simulink model "PSK"  (R2020b)
settings: Solver=VariableStepAuto  StartTime=0.0  StopTime=10.0  RelTol=1e-3
settings Model: Creator=LENOVO  LastModifiedBy=LENOVO

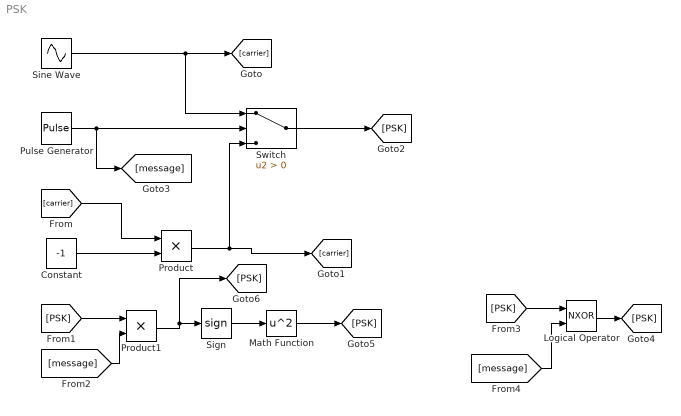
== system PSK ==
  Constant : Constant  Value=-1
  Logical Operator : Logic  Operator=NXOR  AllPortsSameDT=off  OutDataTypeStr=boolean
  Math Function : Math  Operator=square  OutputSignalType=real  SaturateOnIntegerOverflow=on
  Product : Product
  Product1 : Product
  Pulse Generator : DiscretePulseGenerator  PulseType=Time based  Period=10  PulseWidth=5
  Sign : Signum
  Sine Wave : Sin  SampleTime=0
  Switch : Switch  Criteria=u2 > Threshold
  wires:
  Sine Wave/1 -> Switch/1, [carrier]
  Pulse Generator/1 -> [message], Switch/2
  [carrier] -> Product/1
  Constant/1 -> Product/2
  Product/1 -> Switch/3, [carrier]
  [PSK] -> Product1/1
  [message] -> Product1/2
  Switch/1 -> [PSK]
  [PSK] -> Logical Operator/1
  [message] -> Logical Operator/2
  Logical Operator/1 -> [PSK]
  Sign/1 -> Math Function/1
  Product1/1 -> [PSK], Sign/1
  Math Function/1 -> [PSK]
